simulink library "ESSLibrary"  (R2020a)
settings: Solver=VariableStepAuto  StartTime=0.0  StopTime=10.0  RelTol=1e-3
libraries: $bdroot x82, powerlib_meascontrol x10, simulink x7
(part 5 of 7)

== system ESSLibrary/Dispatch/IfActionSubsystem/Subsystem ==
  PSet : Inport
  ChargeEnableSoC : Inport  Port=2
  DischargeEnableSoC : Inport  Port=3
  AND1 : Logic  IconShape=distinctive  AllPortsSameDT=off  OutDataTypeStr=boolean
  AND2 : Logic  IconShape=distinctive  AllPortsSameDT=off  OutDataTypeStr=boolean
  Constant1 : Constant  Value=0  OutDataTypeStr=double
  IsPositive : simulink/Logic and Bit Operations/Compare To Zero  relop=>=  OutDataTypeStr=boolean
  IsPositive1 : simulink/Logic and Bit Operations/Compare To Zero  relop=<=  OutDataTypeStr=boolean
  Switch1 : Switch  Criteria=u2 ~= 0
  Switch2 : Switch  Criteria=u2 ~= 0
  P_Set : Outport
  wires:
  Constant1/1 -> Switch2/3
  PSet/1 -> Switch1/1, Switch2/1, IsPositive1/1, IsPositive/1
  IsPositive/1 -> AND1/1
  DischargeEnableSoC/1 -> AND1/2
  AND1/1 -> Switch1/2
  ChargeEnableSoC/1 -> AND2/2
  IsPositive1/1 -> AND2/1
  AND2/1 -> Switch2/2
  Switch2/1 -> Switch1/3
  Switch1/1 -> P_Set/1

== system ESSLibrary/Divider/IfActionSubsystem/Subsystem ==
  Denominator : Inport  OutDataTypeStr=double
  Compare To Zero : simulink/Logic and Bit Operations/Compare To Zero  relop===  OutDataTypeStr=boolean
  Constant : Constant  Value=0  SampleTime=-1
  Constant3 : Constant  Value=0  SampleTime=-1
  Constant4 : Constant  Value=1000  SampleTime=-1
  Sum : Sum  Inputs=|++
  Switch2 : Switch  Criteria=u2 > Threshold  Threshold=-0.00001
  Switch3 : Switch  Criteria=u2 > Threshold  Threshold=0.00001
  Switch4 : Switch  Criteria=u2 ~= 0
  Divisor : Outport  OutDataTypeStr=double
  Quality : Outport  Port=2  OutDataTypeStr=boolean
  wires:
  Constant4/1 -> Switch4/3
  Switch3/1 -> Sum/1
  Constant3/1 -> Switch2/1
  Sum/1 -> Compare To Zero/1, Switch4/2, Switch4/1
  Denominator/1 -> Switch3/2, Switch3/1, Switch2/2, Switch2/3
  Switch4/1 -> Divisor/1
  Switch2/1 -> Sum/2
  Compare To Zero/1 -> Quality/1
  Constant/1 -> Switch3/3

== system ESSLibrary/DynamicVoltWattMode/MovAvgDeltaVoltCalc/ElseMovAvgFilter ==
  Inp : Inport
  Action Port : ActionPort
  Constant : Constant  Value=0  OutDataTypeStr=int64  SampleTime=-1
  Out : Outport
  ErrorCode : Outport  Port=2
  wires:
  Constant/1 -> ErrorCode/1
  Inp/1 -> Out/1

== system ESSLibrary/DynamicVoltWattMode/MovAvgDeltaVoltCalc/IfMovAvgFilter ==
  Inp : Inport
  FilterTime : Inport  Port=2
  TimeStep : Inport  Port=3
  Action Port : ActionPort
  Constant : Constant  Value=0
  Constant1 : Constant  Value=0
  DiscreteMovingAverage : MATLAB Function  TreatAsAtomicUnit=on
  Enabled Subsystem : Subsystem  TreatAsAtomicUnit=on
  Relational Operator : RelationalOperator  Operator=>  OutDataTypeStr=boolean  ZeroCross=off  RndMeth=Simplest
  Switch : Switch  Criteria=u2 > Threshold
  Out : Outport
  ErrorCode : Outport  Port=2
  wires:
  DiscreteMovingAverage/2(ErrorCode) -> ErrorCode/1
  Constant1/1 -> Switch/3
  DiscreteMovingAverage/1(Out) -> Out/1
  TimeStep/1 -> Relational Operator/1, Enabled Subsystem/1(TimeStep)
  Relational Operator/1 -> Enabled Subsystem/Enable, Switch/2
  Enabled Subsystem/1(NoOfTimeStep) -> Switch/1
  Switch/1 -> DiscreteMovingAverage/1(NoOfTS)
  FilterTime/1 -> Enabled Subsystem/2(FilterTime)
  Constant/1 -> Relational Operator/2
  Inp/1 -> DiscreteMovingAverage/2(Inp)

== system ESSLibrary/FilterResponse/If Action Subsystem/Subsystem1 ==
  Numerator : Inport
  Denominator : Inport  Port=2
  Divide : Product  Inputs=*/
  Subsystem10 : Subsystem
  Quotient : Outport  InitialOutput=0
  Quality : Outport  Port=2  InitialOutput=0
  wires:
  Subsystem10/1(Divisor) -> Divide/2
  Divide/1 -> Quotient/1
  Denominator/1 -> Subsystem10/1(Denominator)
  Numerator/1 -> Divide/1
  Subsystem10/2(Den_Quality) -> Quality/1

== system ESSLibrary/FilterResponse/If Action Subsystem/Subsystem2 ==
  Numerator : Inport
  Denominator : Inport  Port=2
  Divide : Product  Inputs=*/
  Subsystem10 : Subsystem
  Quotient : Outport  InitialOutput=0
  Quality : Outport  Port=2  InitialOutput=0
  wires:
  Subsystem10/2(Den_Quality) -> Quality/1
  Numerator/1 -> Divide/1
  Denominator/1 -> Subsystem10/1(Denominator)
  Divide/1 -> Quotient/1
  Subsystem10/1(Divisor) -> Divide/2

== system ESSLibrary/MovAvgDeltaVoltCalc1/IfMovAvgFilter/Enabled Subsystem ==
  TimeStep : Inport
  FilterTime : Inport  Port=2
  Enable : EnablePort
  Divide : Product  Inputs=*/
  NoOfTimeStep : Outport
  wires:
  Divide/1 -> NoOfTimeStep/1
  TimeStep/1 -> Divide/2
  FilterTime/1 -> Divide/1

== system ESSLibrary/OperationModeSelector/IfAction Subsystem/Comparator ==
  note: LowerThresholdID
  note: UpperThresholdID
  note: CategoryID = 1
  Enable/Disable : Inport
  "Input " : Inport  Port=2
  UpperTrhd : Inport  Port=3
  LowerTrhd : Inport  Port=4
  HystSelection : Inport  Port=5
  AbsHyst : Inport  Port=6
  RelHyst : Inport  Port=7
  VariableIdentifier : Inport  Port=8
  Basic alarm ver2.0 : Subsystem
  CategoryID : Constant  OutDataTypeStr=int64
  Constant1 : Constant  OutDataTypeStr=int64
  Constant10 : Constant  Value=0  OutDataTypeStr=int64
  Constant11 : Constant  Value=0  OutDataTypeStr=int64
  Constant2 : Constant  Value=2  OutDataTypeStr=int64
  Gain : Gain  Gain=100
  Gain1 : Gain  Gain=10000
  Sum : Sum  Inputs=+++  OutDataTypeStr=int64
  Switch1 : Switch  Criteria=u2 ~= 0  OutDataTypeStr=int64
  Switch2 : Switch  Criteria=u2 ~= 0  OutDataTypeStr=int64
  Switch3 : Switch  Criteria=u2 ~= 0  OutDataTypeStr=int64
  Terminator1 : Terminator
  ErrorCode : Outport
  MaxLimitCrossed : Outport  Port=2
  MinLimitCrossed : Outport  Port=3
  wires:
  Basic alarm ver2.0/1(MaxLimitCrossed) -> MaxLimitCrossed/1, Switch1/2
  Constant2/1 -> Switch2/1
  CategoryID/1 -> Gain/1
  Switch1/1 -> Switch3/2, Sum/1
  Constant1/1 -> Switch1/1
  Constant11/1 -> Switch2/3
  HystSelection/1 -> Basic alarm ver2.0/5(HystSelection)
  Basic alarm ver2.0/2(MinLimitCrossed) -> MinLimitCrossed/1, Switch2/2
  Constant10/1 -> Switch3/3
  Basic alarm ver2.0/3(ErrorCode) -> Terminator1/1
  Sum/1 -> Switch3/1
  "Input "/1 -> Basic alarm ver2.0/2("Input ")
  Switch2/1 -> Switch1/3
  VariableIdentifier/1 -> Gain1/1
  AbsHyst/1 -> Basic alarm ver2.0/6(AbsHyst)
  RelHyst/1 -> Basic alarm ver2.0/7(RelHyst)
  Enable/Disable/1 -> Basic alarm ver2.0/1(Enable/disable)
  Switch3/1 -> ErrorCode/1
  UpperTrhd/1 -> Basic alarm ver2.0/3(UpperTrhd)
  LowerTrhd/1 -> Basic alarm ver2.0/4(LowerTrhd)
  Gain/1 -> Sum/2
  Gain1/1 -> Sum/3

== system ESSLibrary/PFReference_P/If Action Subsystem/Basic alarm ver1.0 ==
  Enable/disable : Inport  OutDataTypeStr=boolean
  "Input " : Inport  Port=2
  UpperTrhd : Inport  Port=3
  LowerTrhd : Inport  Port=4
  HystSelection : Inport  Port=5  OutDataTypeStr=int32
  AbsHyst : Inport  Port=6
  RelHyst : Inport  Port=7
  Enable/disable1 : InportShadow  OutDataTypeStr=boolean
  Enabled Subsystem : Subsystem  TreatAsAtomicUnit=on
  Enabled Subsystem1 : Subsystem  TreatAsAtomicUnit=on
  If : If  IfExpression=u1 ~=0
  Switch : Switch  Criteria=u2 > Threshold
  Switch3 : Switch  Criteria=u2 > Threshold
  "Output " : Outport
  ErrorCode : Outport  Port=2
  wires:
  HystSelection/1 -> Enabled Subsystem1/4(HystSelection)
  RelHyst/1 -> Enabled Subsystem1/6(RelHyst)
  AbsHyst/1 -> Enabled Subsystem1/5(AbsHyst)
  LowerTrhd/1 -> Enabled Subsystem1/3(LowerTrhd)
  UpperTrhd/1 -> Enabled Subsystem1/2(UpperTrhd)
  "Input "/1 -> Enabled Subsystem1/1("Input ")
  Enable/disable1/1 -> Switch3/2, Switch/2
  [Else_Logx_value] -> Switch/3
  Switch/1 -> "Output "/1
  Enabled Subsystem1/1("Output ") -> [If_Logx_value]
  [Elase_Errorcode] -> Switch3/3
  [If_Errorcode] -> Switch3/1
  [If_Logx_value] -> Switch/1
  Enabled Subsystem/1("Output ") -> [Else_Logx_value]
  Enabled Subsystem/2(ErrorCode) -> [Elase_Errorcode]
  Switch3/1 -> ErrorCode/1
  Enabled Subsystem1/2(ErrorCode) -> [If_Errorcode]
  If/1 -> Enabled Subsystem1/Action
  If/2 -> Enabled Subsystem/Action
  Enable/disable/1 -> If/1

== system ESSLibrary/PFReference_P/If Action Subsystem/Safe Divider ==
  Enable : Inport  OutDataTypeStr=boolean
  Numerator : Inport  Port=2  OutDataTypeStr=double
  Denominator : Inport  Port=3  OutDataTypeStr=double
  Abs : Abs
  If : If  IfExpression=u1 ~= 0
  Subsystem : Subsystem
  Subsystem1 : Subsystem
  Switch1 : Switch  Criteria=u2 ~= 0
  Switch6 : Switch  Criteria=u2 > Threshold
  Switch7 : Switch  Criteria=u2 > Threshold
  Switch8 : Switch  Criteria=u2 > Threshold
  Quotient : Outport  OutDataTypeStr=double
  Quality : Outport  Port=2  OutDataTypeStr=boolean
  ErrorCode : Outport  Port=3  OutDataTypeStr=int64
  wires:
  If/2 -> Subsystem1/Action
  [Quotient] -> Switch1/2, Switch1/1
  Switch6/1 -> Quality/1
  [DivErrorCode] -> Switch8/1
  Subsystem1/3(Out5) -> [DivErrorCodeD]
  Switch8/1 -> ErrorCode/1
  Subsystem/2(Out) -> [Quotient]
  [QuotientD] -> Switch7/3
  Denominator/1 -> [Denom]
  Switch7/1 -> Quotient/1
  [DivErrorCodeD] -> Switch8/3
  Subsystem1/1(Out3) -> [QualityD]
  Switch1/1 -> Switch7/1
  Subsystem/1(Quality) -> [Quality]
  If/1 -> Subsystem/Action
  Subsystem1/2(Out4) -> [QuotientD]
  [Denom] -> Subsystem/2(Denominator)
  Numerator/1 -> [Num]
  Subsystem/3(ErrorCode) -> [DivErrorCode]
  [Quotient] -> Abs/1
  [Num] -> Subsystem1/1(In1)
  [QualityD] -> Switch6/3
  Enable/1 -> If/1, Switch6/2, Switch7/2, Switch8/2
  Abs/1 -> Switch1/3
  [Num] -> Subsystem/1(Numerator)
  [Quality] -> Switch6/1

== system ESSLibrary/QReference_PF/If Action Subsystem/Subsystem1 ==
  PF : Inport
  PFSign : Inport  Port=2
  PMeas : Inport  Port=3
  Constant : Constant  OutDataTypeStr=boolean
  Constant1 : Constant
  Constant9 : Constant  Value=-1  OutDataTypeStr=double  SampleTime=-1
  Divide : Product  Inputs=**
  Divide3 : Product  Inputs=**
  Safe Divider : Subsystem  Description=|
      | This function divides input values accounting for a predefined dead band for denominator to avoid occurrence of divide by zero condition. 
      | If the input for denominator is inside the dead band then the function returns predefined output with quality bit as one. 
      | If input value for denominator is in the normal range, the function returns the calculated quotient with quality bit as zero.
  Square : Math  Operator=square  SaturateOnIntegerOverflow=on
  Square Root : Sqrt  SaturateOnIntegerOverflow=on
  Sum : Sum  Inputs=+-
  Switch2 : Switch  Criteria=u2 > Threshold
  Terminator2 : Terminator
  QOut : Outport
  ErrorCode : Outport  Port=2
  wires:
  Switch2/1 -> QOut/1
  PMeas/1 -> Divide/1
  Constant9/1 -> Divide3/2
  Safe Divider/1(Quotient) -> Divide/2
  PFSign/1 -> Switch2/2
  Divide/1 -> Divide3/1, Switch2/1
  Square Root/1 -> Safe Divider/2(Numerator)
  Square/1 -> Sum/2
  PF/1 -> Safe Divider/3(Denominator), Square/1
  Sum/1 -> Square Root/1
  Constant1/1 -> Sum/1
  Safe Divider/2(Quality) -> Terminator2/1
  Constant/1 -> Safe Divider/1(Enable)
  Divide3/1 -> Switch2/3
  Safe Divider/3(ErrorCode) -> ErrorCode/1

== system ESSLibrary/SoCManagement/IfActionSubsystem/Comparator ==
  note: CategoryID = 1
  note: UpperThresholdID
  note: LowerThresholdID
  Enable/Disable : Inport
  "Input " : Inport  Port=2
  UpperTrhd : Inport  Port=3
  LowerTrhd : Inport  Port=4
  HystSelection : Inport  Port=5
  AbsHyst : Inport  Port=6
  RelHyst : Inport  Port=7
  VariableIdentifier : Inport  Port=8
  Basic alarm ver2.0 : Subsystem
  CategoryID : Constant  OutDataTypeStr=int64
  Constant1 : Constant  OutDataTypeStr=int64
  Constant10 : Constant  Value=0  OutDataTypeStr=int64
  Constant11 : Constant  Value=0  OutDataTypeStr=int64
  Constant2 : Constant  Value=2  OutDataTypeStr=int64
  Gain : Gain  Gain=100
  Gain1 : Gain  Gain=10000
  Sum : Sum  Inputs=+++  OutDataTypeStr=int64
  Switch1 : Switch  Criteria=u2 ~= 0  OutDataTypeStr=int64
  Switch2 : Switch  Criteria=u2 ~= 0  OutDataTypeStr=int64
  Switch3 : Switch  Criteria=u2 ~= 0  OutDataTypeStr=int64
  Terminator1 : Terminator
  ErrorCode : Outport
  MaxLimitCrossed : Outport  Port=2
  MinLimitCrossed : Outport  Port=3
  wires:
  Gain1/1 -> Sum/3
  Gain/1 -> Sum/2
  LowerTrhd/1 -> Basic alarm ver2.0/4(LowerTrhd)
  UpperTrhd/1 -> Basic alarm ver2.0/3(UpperTrhd)
  Switch3/1 -> ErrorCode/1
  Enable/Disable/1 -> Basic alarm ver2.0/1(Enable/disable)
  RelHyst/1 -> Basic alarm ver2.0/7(RelHyst)
  AbsHyst/1 -> Basic alarm ver2.0/6(AbsHyst)
  VariableIdentifier/1 -> Gain1/1
  Switch2/1 -> Switch1/3
  "Input "/1 -> Basic alarm ver2.0/2("Input ")
  Sum/1 -> Switch3/1
  Basic alarm ver2.0/3(ErrorCode) -> Terminator1/1
  Constant10/1 -> Switch3/3
  Basic alarm ver2.0/2(MinLimitCrossed) -> Switch2/2, MinLimitCrossed/1
  HystSelection/1 -> Basic alarm ver2.0/5(HystSelection)
  Constant11/1 -> Switch2/3
  Constant1/1 -> Switch1/1
  Switch1/1 -> Sum/1, Switch3/2
  CategoryID/1 -> Gain/1
  Constant2/1 -> Switch2/1
  Basic alarm ver2.0/1(MaxLimitCrossed) -> Switch1/2, MaxLimitCrossed/1

== system ESSLibrary/ActivePowerSmoothing/MovAvgDeltaVoltCalc/IfMovAvgFilter/Enabled Subsystem ==
  TimeStep : Inport
  FilterTime : Inport  Port=2
  Enable : EnablePort
  Divide : Product  Inputs=*/
  NoOfTimeStep : Outport
  wires:
  Divide/1 -> NoOfTimeStep/1
  TimeStep/1 -> Divide/2
  FilterTime/1 -> Divide/1

== system ESSLibrary/ChargeDischargeStorageMode/Comparator/Basic alarm ver2.0/Enabled Subsystem ==
  Action Port : ActionPort
  Constant3 : Constant  Value=0  OutDataTypeStr=boolean  SampleTime=-1
  "MaxLimitCrossed " : Outport
  ErrorCode : Outport  Port=2
  MinLimitCrossed : Outport  Port=3
  wires:
  Constant3/1 -> ErrorCode/1, MinLimitCrossed/1, "MaxLimitCrossed "/1

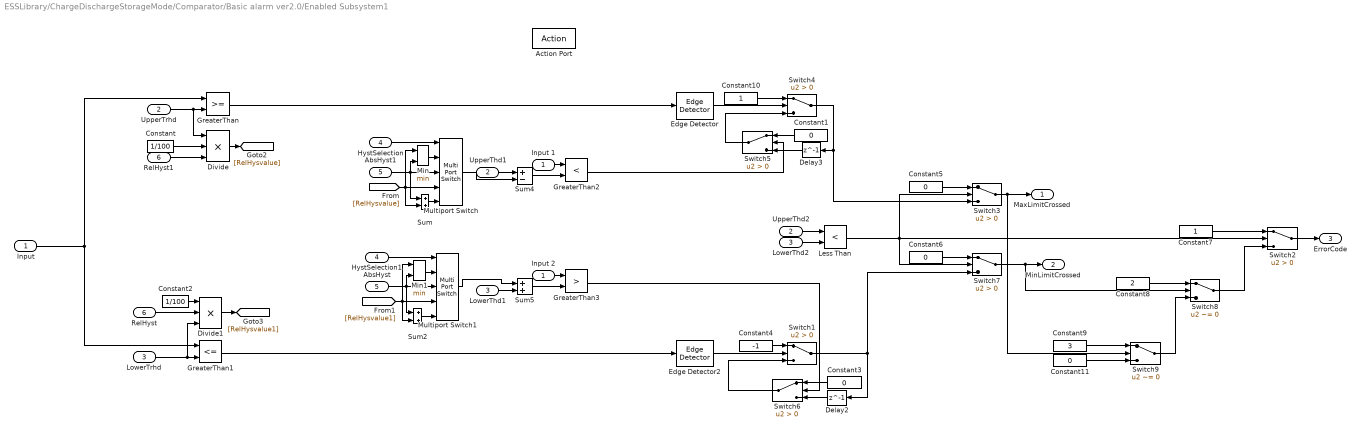
== system ESSLibrary/ChargeDischargeStorageMode/Comparator/Basic alarm ver2.0/Enabled Subsystem1 ==
  "Input " : Inport
  UpperTrhd : Inport  Port=2
  LowerTrhd : Inport  Port=3
  HystSelection : Inport  Port=4
  AbsHyst : Inport  Port=5
  RelHyst : Inport  Port=6
  Action Port : ActionPort
  AbsHyst1 : InportShadow  Port=5
  Constant : Constant  Value=1/100  SampleTime=-1
  Constant1 : Constant  Value=0  OutDataTypeStr=int8  SampleTime=-1
  Constant10 : Constant  OutDataTypeStr=int8  SampleTime=-1
  Constant11 : Constant  Value=0  OutDataTypeStr=int64  SampleTime=-1
  Constant2 : Constant  Value=1/100  SampleTime=-1
  Constant3 : Constant  Value=0  OutDataTypeStr=int8  SampleTime=-1
  Constant4 : Constant  Value=-1  OutDataTypeStr=int8  SampleTime=-1
  Constant5 : Constant  Value=0  OutDataTypeStr=boolean  SampleTime=-1
  Constant6 : Constant  Value=0  OutDataTypeStr=boolean  SampleTime=-1
  Constant7 : Constant  OutDataTypeStr=int64  SampleTime=-1
  Constant8 : Constant  Value=2  OutDataTypeStr=int64  SampleTime=-1
  Constant9 : Constant  Value=3  OutDataTypeStr=int64  SampleTime=-1
  Delay2 : Delay  DelayLength=1  InitialCondition=0
  Delay3 : Delay  DelayLength=1  InitialCondition=0
  Divide : Product  Inputs=***
  Divide1 : Product  Inputs=***
  Edge Detector : powerlib_meascontrol/Logic/Edge Detector  model=Rising  ic=0  Ts=-1
      settings: SourceProductBaseCode=PS
  Edge Detector2 : powerlib_meascontrol/Logic/Edge Detector  model=Rising  ic=0  Ts=-1
      settings: SourceProductBaseCode=PS
  GreaterThan : RelationalOperator  OutDataTypeStr=boolean  RndMeth=Simplest
  GreaterThan1 : RelationalOperator  Operator=<=  OutDataTypeStr=boolean  RndMeth=Simplest
  GreaterThan2 : RelationalOperator  Operator=<  OutDataTypeStr=boolean  RndMeth=Simplest
  GreaterThan3 : RelationalOperator  Operator=>  OutDataTypeStr=boolean  RndMeth=Simplest
  HystSelection1 : InportShadow  Port=4
  Input 1 : InportShadow
  Input 2 : InportShadow
  Less Than : RelationalOperator  Operator=<  OutDataTypeStr=boolean  RndMeth=Simplest
  LowerThd1 : InportShadow  Port=3
  LowerThd2 : InportShadow  Port=3
  Min : MinMax  Inputs=2
  Min1 : MinMax  Inputs=2
  Multiport Switch : MultiPortSwitch  Inputs=4
  Multiport Switch1 : MultiPortSwitch  Inputs=4
  RelHyst1 : InportShadow  Port=6
  Sum : Sum
  Sum2 : Sum
  Sum4 : Sum  Inputs=+-
  Sum5 : Sum
  Switch{1..7} (7 alike) : Switch  Criteria=u2 > Threshold
  Switch8 : Switch  Criteria=u2 ~= 0
  Switch9 : Switch  Criteria=u2 ~= 0
  UpperThd1 : InportShadow  Port=2
  UpperThd2 : InportShadow  Port=2
  MaxLimitCrossed : Outport
  MinLimitCrossed : Outport  Port=2
  ErrorCode : Outport  Port=3  OutDataTypeStr=int64
  wires:
  Constant4/1 -> Switch1/1
  GreaterThan/1 -> Edge Detector/1
  "Input "/1 -> GreaterThan/1, GreaterThan1/1
  UpperTrhd/1 -> Divide/1, GreaterThan/2
  LowerTrhd/1 -> Divide1/3, GreaterThan1/2
  HystSelection/1 -> Multiport Switch/1
  AbsHyst1/1 -> Min/2, Sum/1, Multiport Switch/3
  [RelHysvalue] -> Min/1, Sum/2, Multiport Switch/4
  Sum/1 -> Multiport Switch/5
  Divide/1 -> [RelHysvalue]
  Min/1 -> Multiport Switch/2
  Input 1/1 -> GreaterThan2/1
  Constant10/1 -> Switch4/1
  Edge Detector/1 -> Switch4/2
  Switch5/1 -> Switch4/3
  Switch4/1 -> Switch3/3, Delay3/1
  Constant/1 -> Divide/2
  RelHyst1/1 -> Divide/3
  RelHyst/1 -> Divide1/2
  Constant2/1 -> Divide1/1
  Divide1/1 -> [RelHysvalue1]
  HystSelection1/1 -> Multiport Switch1/1
  Min1/1 -> Multiport Switch1/2
  AbsHyst/1 -> Sum2/1, Min1/2, Multiport Switch1/3
  [RelHysvalue1] -> Sum2/2, Multiport Switch1/4, Min1/1
  Sum2/1 -> Multiport Switch1/5
  Input 2/1 -> GreaterThan3/1
  GreaterThan1/1 -> Edge Detector2/1
  Edge Detector2/1 -> Switch1/2
  Switch6/1 -> Switch1/3
  GreaterThan3/1 -> Switch6/2
  Sum4/1 -> GreaterThan2/2
  Multiport Switch/1 -> Sum4/2
  UpperThd1/1 -> Sum4/1
  Sum5/1 -> GreaterThan3/2
  Multiport Switch1/1 -> Sum5/1
  LowerThd1/1 -> Sum5/2
  GreaterThan2/1 -> Switch5/2
  Constant1/1 -> Switch5/1
  Constant3/1 -> Switch6/1
  Delay3/1 -> Switch5/3
  Delay2/1 -> Switch6/3
  Switch3/1 -> Switch9/2, MaxLimitCrossed/1
  Less Than/1 -> Switch2/2, Switch3/2, Switch7/2
  Constant5/1 -> Switch3/1
  Switch1/1 -> Switch7/3, Delay2/1
  Constant6/1 -> Switch7/1
  Switch7/1 -> Switch8/2, MinLimitCrossed/1
  Switch8/1 -> Switch2/3
  Constant7/1 -> Switch2/1
  Switch2/1 -> ErrorCode/1
  LowerThd2/1 -> Less Than/2
  UpperThd2/1 -> Less Than/1
  Constant8/1 -> Switch8/1
  Constant9/1 -> Switch9/1
  Constant11/1 -> Switch9/3
  Switch9/1 -> Switch8/3

== system ESSLibrary/Dispatch/IfActionSubsystem/PrioritySelector/ActivePowerPriority ==
  "EnablePQCapabilityCurve " : Inport
  Pcapability1 : Inport  Port=2
  Pcapability2 : Inport  Port=3
  Pcapability3 : Inport  Port=4
  Pcapability4 : Inport  Port=5
  Pcapability5 : Inport  Port=6
  Pcapability6 : Inport  Port=7
  Pcapability7 : Inport  Port=8
  Pcapability8 : Inport  Port=9
  Qcapability1 : Inport  Port=10
  Qcapability2 : Inport  Port=11
  Qcapability3 : Inport  Port=12
  Qcapability4 : Inport  Port=13
  Qcapability5 : Inport  Port=14
  Qcapability6 : Inport  Port=15
  Qcapability7 : Inport  Port=16
  Qcapability8 : Inport  Port=17
  ECPAppPow : Inport  Port=18
  EnablePFLimit : Inport  Port=19
  PFOperMax : Inport  Port=20
  PFOperMin : Inport  Port=21
  ActivePowerCalc : Inport  Port=22
  ReactivePowerCalc : Inport  Port=23
  Action Port : ActionPort  ActionPortLabel=else
  ActivePowerCalc1 : InportShadow  Port=22
  ActivePowerPriority_NoPQCurve : Subsystem  TreatAsAtomicUnit=on
  ActivePowerPriority_PQCurve : Subsystem  TreatAsAtomicUnit=on
  ECPAppPow1 : InportShadow  Port=18
  EnablePFLimit1 : InportShadow  Port=19
  If : If  IfExpression=u1 == 1
  Merge : Merge
  Merge1 : Merge
  PFOperMax1 : InportShadow  Port=20
  PFOperMin1 : InportShadow  Port=21
  ReactivePowerCalc1 : InportShadow  Port=23
  ActivePowerOut : Outport
  ReactivePowerOut : Outport  Port=2
  wires:
  "EnablePQCapabilityCurve "/1 -> If/1
  If/1 -> ActivePowerPriority_PQCurve/Action
  If/2 -> ActivePowerPriority_NoPQCurve/Action
  Pcapability1/1 -> ActivePowerPriority_PQCurve/1(Pcapability1)
  Pcapability2/1 -> ActivePowerPriority_PQCurve/2(Pcapability2)
  Pcapability3/1 -> ActivePowerPriority_PQCurve/3(Pcapability3)
  Pcapability4/1 -> ActivePowerPriority_PQCurve/4(Pcapability4)
  Pcapability5/1 -> ActivePowerPriority_PQCurve/5(Pcapability5)
  Pcapability6/1 -> ActivePowerPriority_PQCurve/6(Pcapability6)
  Pcapability7/1 -> ActivePowerPriority_PQCurve/7(Pcapability7)
  Pcapability8/1 -> ActivePowerPriority_PQCurve/8(Pcapability8)
  Qcapability1/1 -> ActivePowerPriority_PQCurve/9(Qcapability1)
  Qcapability2/1 -> ActivePowerPriority_PQCurve/10(Qcapability2)
  Qcapability3/1 -> ActivePowerPriority_PQCurve/11(Qcapability3)
  Qcapability4/1 -> ActivePowerPriority_PQCurve/12(Qcapability4)
  Qcapability5/1 -> ActivePowerPriority_PQCurve/13(Qcapability5)
  Qcapability6/1 -> ActivePowerPriority_PQCurve/14(Qcapability6)
  Qcapability7/1 -> ActivePowerPriority_PQCurve/15(Qcapability7)
  Qcapability8/1 -> ActivePowerPriority_PQCurve/16(Qcapability8)
  ECPAppPow/1 -> ActivePowerPriority_PQCurve/17(ECPAppPow)
  EnablePFLimit/1 -> ActivePowerPriority_PQCurve/18(EnablePFLimit)
  PFOperMax/1 -> ActivePowerPriority_PQCurve/19(PFOperMax)
  PFOperMin/1 -> ActivePowerPriority_PQCurve/20(PFOperMin)
  ActivePowerCalc/1 -> ActivePowerPriority_PQCurve/21(ActivePowerCalc)
  ReactivePowerCalc/1 -> ActivePowerPriority_PQCurve/22(ReactivePowerCalc)
  ActivePowerPriority_NoPQCurve/1(ActivePowerOut) -> [ActivePowerPriority_NoPQCurveActivePowerOut]
  ActivePowerPriority_NoPQCurve/2(ReactivePowerOut) -> [ActivePowerPriority_NoPQCurveReactivePowerOut]
  ActivePowerPriority_PQCurve/1(ActivePowerOut) -> [ActivePowerPriority_PQCurveActivePowerOut]
  ActivePowerPriority_PQCurve/2(ReactivePowerOut) -> [ActivePowerPriority_PQCurveReactivePowerOut]
  [ActivePowerPriority_NoPQCurveActivePowerOut] -> Merge/1
  [ActivePowerPriority_PQCurveActivePowerOut] -> Merge/2
  [ActivePowerPriority_NoPQCurveReactivePowerOut] -> Merge1/1
  [ActivePowerPriority_PQCurveReactivePowerOut] -> Merge1/2
  Merge/1 -> ActivePowerOut/1
  Merge1/1 -> ReactivePowerOut/1
  ActivePowerCalc1/1 -> ActivePowerPriority_NoPQCurve/1(ActivePowerCalc)
  ECPAppPow1/1 -> ActivePowerPriority_NoPQCurve/3(ECPAppPow)
  ReactivePowerCalc1/1 -> ActivePowerPriority_NoPQCurve/2(ReactivePowerCalc)
  EnablePFLimit1/1 -> ActivePowerPriority_NoPQCurve/4(EnablePFLimit)
  PFOperMax1/1 -> ActivePowerPriority_NoPQCurve/5(PFOperMax)
  PFOperMin1/1 -> ActivePowerPriority_NoPQCurve/6(PFOperMin)

== system ESSLibrary/Dispatch/IfActionSubsystem/PrioritySelector/ReactivePowerPriority ==
  "EnablePQCapabilityCurve " : Inport
  Pcapability1 : Inport  Port=2
  Pcapability2 : Inport  Port=3
  Pcapability3 : Inport  Port=4
  Pcapability4 : Inport  Port=5
  Pcapability5 : Inport  Port=6
  Pcapability6 : Inport  Port=7
  Pcapability7 : Inport  Port=8
  Pcapability8 : Inport  Port=9
  Qcapability1 : Inport  Port=10
  Qcapability2 : Inport  Port=11
  Qcapability3 : Inport  Port=12
  Qcapability4 : Inport  Port=13
  Qcapability5 : Inport  Port=14
  Qcapability6 : Inport  Port=15
  Qcapability7 : Inport  Port=16
  Qcapability8 : Inport  Port=17
  ECPAppPow : Inport  Port=18
  EnablePFLimit : Inport  Port=19
  PFOperMax : Inport  Port=20
  PFOperMin : Inport  Port=21
  ActivePowerCalc : Inport  Port=22
  ReactivePowerCalc : Inport  Port=23
  Action Port : ActionPort  ActionPortLabel=if(u1 == 2)
  ActivePowerCalc1 : InportShadow  Port=22
  ECPAppPow1 : InportShadow  Port=18
  EnablePFLimit1 : InportShadow  Port=19
  If : If  IfExpression=u1 == 1
  Merge : Merge
  Merge1 : Merge
  PFOperMax1 : InportShadow  Port=20
  PFOperMin1 : InportShadow  Port=21
  ReactivePowerCalc1 : InportShadow  Port=23
  ReactivePowerPriority_NoPQCurve : Subsystem  TreatAsAtomicUnit=on
  ReactivePowerPriority_PQCurve : Subsystem  TreatAsAtomicUnit=on
  ActivePowerOut : Outport
  ReactivePowerOut : Outport  Port=2
  wires:
  "EnablePQCapabilityCurve "/1 -> If/1
  If/1 -> ReactivePowerPriority_PQCurve/Action
  If/2 -> ReactivePowerPriority_NoPQCurve/Action
  Pcapability1/1 -> ReactivePowerPriority_PQCurve/1(Pcapability1)
  Pcapability2/1 -> ReactivePowerPriority_PQCurve/2(Pcapability2)
  Pcapability3/1 -> ReactivePowerPriority_PQCurve/3(Pcapability3)
  Pcapability4/1 -> ReactivePowerPriority_PQCurve/4(Pcapability4)
  Pcapability5/1 -> ReactivePowerPriority_PQCurve/5(Pcapability5)
  Pcapability6/1 -> ReactivePowerPriority_PQCurve/6(Pcapability6)
  Pcapability7/1 -> ReactivePowerPriority_PQCurve/7(Pcapability7)
  Pcapability8/1 -> ReactivePowerPriority_PQCurve/8(Pcapability8)
  Qcapability1/1 -> ReactivePowerPriority_PQCurve/9(Qcapability1)
  Qcapability2/1 -> ReactivePowerPriority_PQCurve/10(Qcapability2)
  Qcapability3/1 -> ReactivePowerPriority_PQCurve/11(Qcapability3)
  Qcapability4/1 -> ReactivePowerPriority_PQCurve/12(Qcapability4)
  Qcapability5/1 -> ReactivePowerPriority_PQCurve/13(Qcapability5)
  Qcapability6/1 -> ReactivePowerPriority_PQCurve/14(Qcapability6)
  Qcapability7/1 -> ReactivePowerPriority_PQCurve/15(Qcapability7)
  Qcapability8/1 -> ReactivePowerPriority_PQCurve/16(Qcapability8)
  ECPAppPow/1 -> ReactivePowerPriority_PQCurve/17(ECPAppPow)
  EnablePFLimit/1 -> ReactivePowerPriority_PQCurve/18(EnablePFLimit)
  PFOperMax/1 -> ReactivePowerPriority_PQCurve/19(PFOperMax)
  PFOperMin/1 -> ReactivePowerPriority_PQCurve/20(PFOperMin)
  ActivePowerCalc/1 -> ReactivePowerPriority_PQCurve/21(ActivePowerCalc)
  ReactivePowerCalc/1 -> ReactivePowerPriority_PQCurve/22(ReactivePowerCalc)
  ReactivePowerPriority_NoPQCurve/1(ActivePowerOut) -> [ActivePowerPriority_NoPQCurveActivePowerOut]
  ReactivePowerPriority_NoPQCurve/2(ReactivePowerOut) -> [ActivePowerPriority_NoPQCurveReactivePowerOut]
  ReactivePowerPriority_PQCurve/1(ActivePowerOut) -> [ActivePowerPriority_PQCurveActivePowerOut]
  ReactivePowerPriority_PQCurve/2(ReactivePowerOut) -> [ActivePowerPriority_PQCurveReactivePowerOut]
  [ActivePowerPriority_NoPQCurveActivePowerOut] -> Merge/1
  [ActivePowerPriority_PQCurveActivePowerOut] -> Merge/2
  [ActivePowerPriority_NoPQCurveReactivePowerOut] -> Merge1/1
  [ActivePowerPriority_PQCurveReactivePowerOut] -> Merge1/2
  Merge/1 -> ActivePowerOut/1
  Merge1/1 -> ReactivePowerOut/1
  ActivePowerCalc1/1 -> ReactivePowerPriority_NoPQCurve/1(ActivePowerCalc)
  ECPAppPow1/1 -> ReactivePowerPriority_NoPQCurve/3(ECPAppPow)
  ReactivePowerCalc1/1 -> ReactivePowerPriority_NoPQCurve/2(ReactivePowerCalc)
  EnablePFLimit1/1 -> ReactivePowerPriority_NoPQCurve/4(EnablePFLimit)
  PFOperMax1/1 -> ReactivePowerPriority_NoPQCurve/5(PFOperMax)
  PFOperMin1/1 -> ReactivePowerPriority_NoPQCurve/6(PFOperMin)

== system ESSLibrary/DynamicVoltWattMode/MovAvgDeltaVoltCalc/IfMovAvgFilter/Enabled Subsystem ==
  TimeStep : Inport
  FilterTime : Inport  Port=2
  Enable : EnablePort
  Divide : Product  Inputs=*/
  NoOfTimeStep : Outport
  wires:
  FilterTime/1 -> Divide/1
  TimeStep/1 -> Divide/2
  Divide/1 -> NoOfTimeStep/1

== system ESSLibrary/FilterResponse/If Action Subsystem/Subsystem1/Subsystem10 ==
  Denominator : Inport
  Compare To Zero : simulink/Logic and Bit Operations/Compare To Zero  relop===  OutDataTypeStr=boolean
  Constant4 : Constant  SampleTime=-1
  Switch3 : Switch  Criteria=u2 ~= 0
  Divisor : Outport
  Den_Quality : Outport  Port=2
  wires:
  Denominator/1 -> Switch3/1, Switch3/2, Compare To Zero/1
  Switch3/1 -> Divisor/1
  Compare To Zero/1 -> Den_Quality/1
  Constant4/1 -> Switch3/3

== system ESSLibrary/FilterResponse/If Action Subsystem/Subsystem2/Subsystem10 ==
  Denominator : Inport
  Compare To Zero : simulink/Logic and Bit Operations/Compare To Zero  relop===  OutDataTypeStr=boolean
  Constant4 : Constant  SampleTime=-1
  Switch3 : Switch  Criteria=u2 ~= 0
  Divisor : Outport
  Den_Quality : Outport  Port=2
  wires:
  Constant4/1 -> Switch3/3
  Compare To Zero/1 -> Den_Quality/1
  Switch3/1 -> Divisor/1
  Denominator/1 -> Compare To Zero/1, Switch3/2, Switch3/1

== system ESSLibrary/OperationModeSelector/IfAction Subsystem/Comparator/Basic alarm ver2.0 ==
  Enable/disable : Inport  OutDataTypeStr=boolean
  "Input " : Inport  Port=2
  UpperTrhd : Inport  Port=3
  LowerTrhd : Inport  Port=4
  HystSelection : Inport  Port=5  OutDataTypeStr=int32
  AbsHyst : Inport  Port=6
  RelHyst : Inport  Port=7
  Enable/disable1 : InportShadow  OutDataTypeStr=boolean
  Enabled Subsystem : Subsystem  TreatAsAtomicUnit=on
  Enabled Subsystem1 : Subsystem  TreatAsAtomicUnit=on
  If : If  IfExpression=u1 ~=0
  Switch : Switch  Criteria=u2 > Threshold
  Switch1 : Switch  Criteria=u2 > Threshold
  Switch3 : Switch  Criteria=u2 > Threshold
  MaxLimitCrossed : Outport  OutDataTypeStr=boolean
  MinLimitCrossed : Outport  Port=2  OutDataTypeStr=boolean
  ErrorCode : Outport  Port=3  OutDataTypeStr=int64
  wires:
  Enable/disable/1 -> If/1
  If/2 -> Enabled Subsystem/Action
  If/1 -> Enabled Subsystem1/Action
  Enabled Subsystem1/3(ErrorCode) -> [If_Errorcode]
  Enabled Subsystem/2(ErrorCode) -> [Else_Errorcode]
  Enabled Subsystem/1("MaxLimitCrossed ") -> [Else_MaxLimitCrossed]
  [If_MaxLimitCrossed] -> Switch/1
  [If_Errorcode] -> Switch3/1
  [Else_Errorcode] -> Switch3/3
  Enabled Subsystem1/1(MaxLimitCrossed) -> [If_MaxLimitCrossed]
  Switch/1 -> MaxLimitCrossed/1
  [Else_MaxLimitCrossed] -> Switch/3
  Enable/disable1/1 -> Switch3/2, Switch1/2, Switch/2
  "Input "/1 -> Enabled Subsystem1/1("Input ")
  UpperTrhd/1 -> Enabled Subsystem1/2(UpperTrhd)
  LowerTrhd/1 -> Enabled Subsystem1/3(LowerTrhd)
  AbsHyst/1 -> Enabled Subsystem1/5(AbsHyst)
  RelHyst/1 -> Enabled Subsystem1/6(RelHyst)
  HystSelection/1 -> Enabled Subsystem1/4(HystSelection)
  Enabled Subsystem1/2(MinLimitCrossed) -> [If_MinLimitCrossed]
  Enabled Subsystem/3(MinLimitCrossed) -> [Else_MinLimitCrossed]
  [If_MinLimitCrossed] -> Switch1/1
  [Else_MinLimitCrossed] -> Switch1/3
  Switch1/1 -> MinLimitCrossed/1
  Switch3/1 -> ErrorCode/1

== system ESSLibrary/PFReference_P/If Action Subsystem/Basic alarm ver1.0/Enabled Subsystem ==
  Action Port : ActionPort
  Constant2 : Constant  Value=00000000000009  OutDataTypeStr=int32
  Constant3 : Constant  Value=0  OutDataTypeStr=double
  "Output " : Outport
  ErrorCode : Outport  Port=2
  wires:
  Constant3/1 -> "Output "/1
  Constant2/1 -> ErrorCode/1

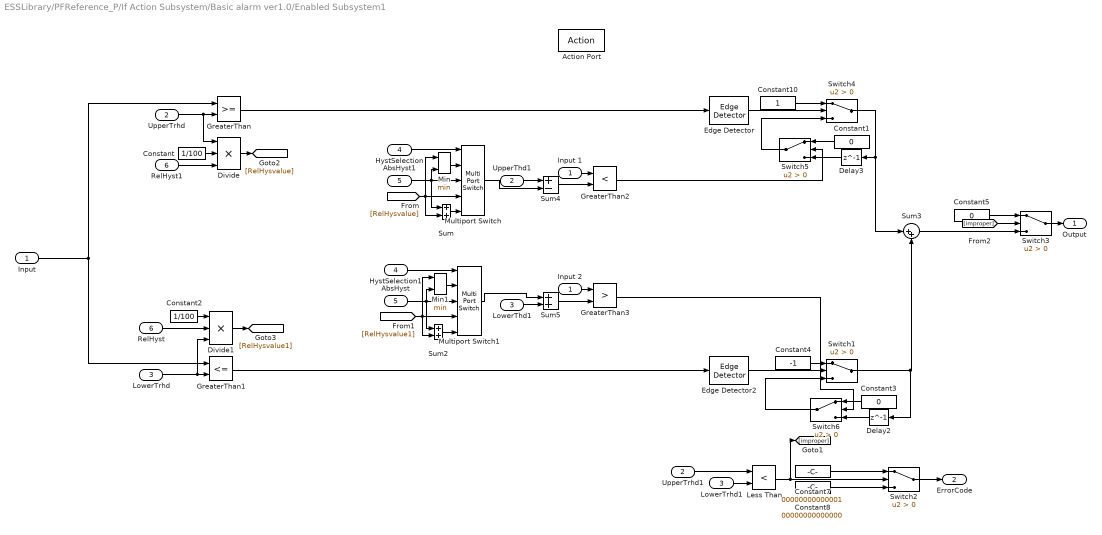
== system ESSLibrary/PFReference_P/If Action Subsystem/Basic alarm ver1.0/Enabled Subsystem1 ==
  "Input " : Inport
  UpperTrhd : Inport  Port=2
  LowerTrhd : Inport  Port=3
  HystSelection : Inport  Port=4
  AbsHyst : Inport  Port=5
  RelHyst : Inport  Port=6
  Action Port : ActionPort
  AbsHyst1 : InportShadow  Port=5
  Constant : Constant  Value=1/100  SampleTime=-1
  Constant1 : Constant  Value=0  OutDataTypeStr=int32  SampleTime=-1
  Constant10 : Constant  OutDataTypeStr=int32  SampleTime=-1
  Constant2 : Constant  Value=1/100  SampleTime=-1
  Constant3 : Constant  Value=0  OutDataTypeStr=int32  SampleTime=-1
  Constant4 : Constant  Value=-1  OutDataTypeStr=int32  SampleTime=-1
  Constant5 : Constant  Value=0  OutDataTypeStr=int32  SampleTime=-1
  Constant7 : Constant  Value=00000000000001  OutDataTypeStr=int32  SampleTime=-1
  Constant8 : Constant  Value=00000000000000  OutDataTypeStr=int32  SampleTime=-1
  Delay2 : Delay  DelayLength=1  InitialCondition=0
  Delay3 : Delay  DelayLength=1  InitialCondition=0
  Divide : Product  Inputs=***
  Divide1 : Product  Inputs=***
  Edge Detector : powerlib_meascontrol/Logic/Edge Detector  model=Rising  ic=0  Ts=-1
      settings: SourceProductBaseCode=PS
  Edge Detector2 : powerlib_meascontrol/Logic/Edge Detector  model=Rising  ic=0  Ts=-1
      settings: SourceProductBaseCode=PS
  GreaterThan : RelationalOperator  OutDataTypeStr=boolean  RndMeth=Simplest
  GreaterThan1 : RelationalOperator  Operator=<=  OutDataTypeStr=boolean  RndMeth=Simplest
  GreaterThan2 : RelationalOperator  Operator=<  OutDataTypeStr=boolean  RndMeth=Simplest
  GreaterThan3 : RelationalOperator  Operator=>  OutDataTypeStr=boolean  RndMeth=Simplest
  HystSelection1 : InportShadow  Port=4
  Input 1 : InportShadow
  Input 2 : InportShadow
  Less Than : RelationalOperator  Operator=<  OutDataTypeStr=boolean  RndMeth=Simplest
  LowerThd1 : InportShadow  Port=3
  LowerTrhd1 : InportShadow  Port=3
  Min : MinMax  Inputs=2
  Min1 : MinMax  Inputs=2
  Multiport Switch : MultiPortSwitch  Inputs=4
  Multiport Switch1 : MultiPortSwitch  Inputs=4
  RelHyst1 : InportShadow  Port=6
  Sum : Sum
  Sum2 : Sum
  Sum3 : Sum  Inputs=|++
  Sum4 : Sum  Inputs=+-
  Sum5 : Sum
  Switch{1..6} (6 alike) : Switch  Criteria=u2 > Threshold
  UpperThd1 : InportShadow  Port=2
  UpperTrhd1 : InportShadow  Port=2
  "Output " : Outport
  ErrorCode : Outport  Port=2
  wires:
  Sum3/1 -> Switch3/3
  Constant5/1 -> Switch3/1
  [improper] -> Switch3/2
  Switch3/1 -> "Output "/1
  LowerTrhd1/1 -> Less Than/2
  UpperTrhd1/1 -> Less Than/1
  Delay2/1 -> Switch6/3
  Delay3/1 -> Switch5/3
  Constant3/1 -> Switch6/1
  Constant1/1 -> Switch5/1
  GreaterThan2/1 -> Switch5/2
  LowerThd1/1 -> Sum5/2
  Multiport Switch1/1 -> Sum5/1
  Sum5/1 -> GreaterThan3/2
  UpperThd1/1 -> Sum4/1
  Multiport Switch/1 -> Sum4/2
  Sum4/1 -> GreaterThan2/2
  Switch1/1 -> Sum3/2, Delay2/1
  GreaterThan3/1 -> Switch6/2
  Switch6/1 -> Switch1/3
  Edge Detector2/1 -> Switch1/2
  GreaterThan1/1 -> Edge Detector2/1
  Input 2/1 -> GreaterThan3/1
  Sum2/1 -> Multiport Switch1/5
  [RelHysvalue1] -> Min1/1, Multiport Switch1/4, Sum2/2
  AbsHyst/1 -> Multiport Switch1/3, Min1/2, Sum2/1
  Min1/1 -> Multiport Switch1/2
  HystSelection1/1 -> Multiport Switch1/1
  Divide1/1 -> [RelHysvalue1]
  Constant2/1 -> Divide1/1
  RelHyst/1 -> Divide1/2
  RelHyst1/1 -> Divide/3
  Constant/1 -> Divide/2
  Switch4/1 -> Sum3/1, Delay3/1
  Switch5/1 -> Switch4/3
  Edge Detector/1 -> Switch4/2
  Constant10/1 -> Switch4/1
  Input 1/1 -> GreaterThan2/1
  Min/1 -> Multiport Switch/2
  Divide/1 -> [RelHysvalue]
  Sum/1 -> Multiport Switch/5
  [RelHysvalue] -> Multiport Switch/4, Sum/2, Min/1
  AbsHyst1/1 -> Multiport Switch/3, Sum/1, Min/2
  HystSelection/1 -> Multiport Switch/1
  LowerTrhd/1 -> GreaterThan1/2, Divide1/3
  UpperTrhd/1 -> GreaterThan/2, Divide/1
  "Input "/1 -> GreaterThan1/1, GreaterThan/1
  GreaterThan/1 -> Edge Detector/1
  Constant4/1 -> Switch1/1
  Constant7/1 -> Switch2/1
  Constant8/1 -> Switch2/3
  Less Than/1 -> Switch2/2, [improper]
  Switch2/1 -> ErrorCode/1

== system ESSLibrary/PFReference_P/If Action Subsystem/Safe Divider/Subsystem ==
  Numerator : Inport  OutDataTypeStr=double
  Denominator : Inport  Port=2  OutDataTypeStr=double
  Action Port : ActionPort
  Constant1 : Constant  OutDataTypeStr=int64  SampleTime=-1
  Constant11 : Constant  SampleTime=-1
  Constant2 : Constant  Value=0  OutDataTypeStr=int64  SampleTime=-1
  Divide8 : Product  Inputs=*/
  NOT : Logic  Operator=NOT  IconShape=distinctive  AllPortsSameDT=off  OutDataTypeStr=boolean
  NOT1 : Logic  Operator=NOT  IconShape=distinctive  AllPortsSameDT=off  OutDataTypeStr=boolean
  Subsystem21 : Subsystem
  Switch1 : Switch  Criteria=u2 ~= 0
  Switch11 : Switch  Criteria=u2 ~= 0
  Quality : Outport  OutDataTypeStr=boolean
  Out : Outport  Port=2  OutDataTypeStr=double
  ErrorCode : Outport  Port=3  OutDataTypeStr=int64
  wires:
  [Quality2] -> Quality/1
  Constant2/1 -> Switch1/1
  Switch11/1 -> Out/1
  Subsystem21/2(Quality) -> [Quality2]
  Constant11/1 -> Switch11/3
  Subsystem21/1(Divisor) -> [Divisor]
  Numerator/1 -> Divide8/1
  Divide8/1 -> Switch11/1
  [Quality2] -> NOT/1
  [Divisor] -> Divide8/2
  Denominator/1 -> Subsystem21/1(Denominator)
  Constant1/1 -> Switch1/3
  Switch1/1 -> ErrorCode/1
  [Quality2] -> NOT1/1
  NOT/1 -> Switch11/2
  NOT1/1 -> Switch1/2

== system ESSLibrary/PFReference_P/If Action Subsystem/Safe Divider/Subsystem1 ==
  In1 : Inport  OutDataTypeStr=double
  Action Port : ActionPort
  Constant1 : Constant  Value=9  OutDataTypeStr=int64  SampleTime=-1
  Constant11 : Constant  Value=0  OutDataTypeStr=boolean  SampleTime=-1
  Out3 : Outport  OutDataTypeStr=boolean
  Out4 : Outport  Port=2  OutDataTypeStr=double
  Out5 : Outport  Port=3  OutDataTypeStr=int64
  wires:
  Constant1/1 -> Out5/1
  Constant11/1 -> Out3/1
  In1/1 -> Out4/1

== system ESSLibrary/QReference_PF/If Action Subsystem/Subsystem1/Safe Divider ==
  Enable : Inport  OutDataTypeStr=boolean
  Numerator : Inport  Port=2  OutDataTypeStr=double
  Denominator : Inport  Port=3  OutDataTypeStr=double
  Abs : Abs
  If : If  IfExpression=u1 ~= 0
  Subsystem : Subsystem
  Subsystem1 : Subsystem
  Switch1 : Switch  Criteria=u2 ~= 0
  Switch6 : Switch  Criteria=u2 > Threshold
  Switch7 : Switch  Criteria=u2 > Threshold
  Switch8 : Switch  Criteria=u2 > Threshold
  Quotient : Outport  OutDataTypeStr=double
  Quality : Outport  Port=2  OutDataTypeStr=boolean
  ErrorCode : Outport  Port=3  OutDataTypeStr=int64
  wires:
  If/2 -> Subsystem1/Action
  [Quotient] -> Switch1/2, Switch1/1
  Switch6/1 -> Quality/1
  [DivErrorCode] -> Switch8/1
  Subsystem1/3(Out5) -> [DivErrorCodeD]
  Switch8/1 -> ErrorCode/1
  Subsystem/2(Out) -> [Quotient]
  [QuotientD] -> Switch7/3
  Denominator/1 -> [Denom]
  Switch7/1 -> Quotient/1
  [DivErrorCodeD] -> Switch8/3
  Subsystem1/1(Out3) -> [QualityD]
  Switch1/1 -> Switch7/1
  Subsystem/1(Quality) -> [Quality]
  If/1 -> Subsystem/Action
  Subsystem1/2(Out4) -> [QuotientD]
  [Denom] -> Subsystem/2(Denominator)
  Numerator/1 -> [Num]
  Subsystem/3(ErrorCode) -> [DivErrorCode]
  [Quotient] -> Abs/1
  [Num] -> Subsystem1/1(In1)
  [QualityD] -> Switch6/3
  Enable/1 -> If/1, Switch6/2, Switch7/2, Switch8/2
  Abs/1 -> Switch1/3
  [Num] -> Subsystem/1(Numerator)
  [Quality] -> Switch6/1

== system ESSLibrary/SoCManagement/IfActionSubsystem/Comparator/Basic alarm ver2.0 ==
  Enable/disable : Inport  OutDataTypeStr=boolean
  "Input " : Inport  Port=2
  UpperTrhd : Inport  Port=3
  LowerTrhd : Inport  Port=4
  HystSelection : Inport  Port=5  OutDataTypeStr=int32
  AbsHyst : Inport  Port=6
  RelHyst : Inport  Port=7
  Enable/disable1 : InportShadow  OutDataTypeStr=boolean
  Enabled Subsystem : Subsystem  TreatAsAtomicUnit=on
  Enabled Subsystem1 : Subsystem  TreatAsAtomicUnit=on
  If : If  IfExpression=u1 ~=0
  Switch : Switch  Criteria=u2 > Threshold
  Switch1 : Switch  Criteria=u2 > Threshold
  Switch3 : Switch  Criteria=u2 > Threshold
  MaxLimitCrossed : Outport  OutDataTypeStr=boolean
  MinLimitCrossed : Outport  Port=2  OutDataTypeStr=boolean
  ErrorCode : Outport  Port=3  OutDataTypeStr=int64
  wires:
  Switch3/1 -> ErrorCode/1
  Switch1/1 -> MinLimitCrossed/1
  [Else_MinLimitCrossed] -> Switch1/3
  [If_MinLimitCrossed] -> Switch1/1
  Enabled Subsystem/3(MinLimitCrossed) -> [Else_MinLimitCrossed]
  Enabled Subsystem1/2(MinLimitCrossed) -> [If_MinLimitCrossed]
  HystSelection/1 -> Enabled Subsystem1/4(HystSelection)
  RelHyst/1 -> Enabled Subsystem1/6(RelHyst)
  AbsHyst/1 -> Enabled Subsystem1/5(AbsHyst)
  LowerTrhd/1 -> Enabled Subsystem1/3(LowerTrhd)
  UpperTrhd/1 -> Enabled Subsystem1/2(UpperTrhd)
  "Input "/1 -> Enabled Subsystem1/1("Input ")
  Enable/disable1/1 -> Switch/2, Switch1/2, Switch3/2
  [Else_MaxLimitCrossed] -> Switch/3
  Switch/1 -> MaxLimitCrossed/1
  Enabled Subsystem1/1(MaxLimitCrossed) -> [If_MaxLimitCrossed]
  [Else_Errorcode] -> Switch3/3
  [If_Errorcode] -> Switch3/1
  [If_MaxLimitCrossed] -> Switch/1
  Enabled Subsystem/1("MaxLimitCrossed ") -> [Else_MaxLimitCrossed]
  Enabled Subsystem/2(ErrorCode) -> [Else_Errorcode]
  Enabled Subsystem1/3(ErrorCode) -> [If_Errorcode]
  If/1 -> Enabled Subsystem1/Action
  If/2 -> Enabled Subsystem/Action
  Enable/disable/1 -> If/1

== system ESSLibrary/Dispatch/IfActionSubsystem/PrioritySelector/ActivePowerPriority/ActivePowerPriority_NoPQCurve ==
  ActivePowerCalc : Inport
  ReactivePowerCalc : Inport  Port=2
  ECPAppPow : Inport  Port=3
  EnablePFLimit : Inport  Port=4
  PFOperMax : Inport  Port=5
  PFOperMin : Inport  Port=6
  Action Port : ActionPort  ActionPortLabel=else
  ActivePowerPriority_NoPQCurve : MATLAB Function  TreatAsAtomicUnit=on
  ActivePowerOut : Outport
  ReactivePowerOut : Outport  Port=2
  wires:
  ActivePowerCalc/1 -> ActivePowerPriority_NoPQCurve/1(ActivePowerCalc)
  ReactivePowerCalc/1 -> ActivePowerPriority_NoPQCurve/2(ReactivePowerCalc)
  ECPAppPow/1 -> ActivePowerPriority_NoPQCurve/3(ECPAppPow)
  EnablePFLimit/1 -> ActivePowerPriority_NoPQCurve/4(EnablePFLimit)
  PFOperMax/1 -> ActivePowerPriority_NoPQCurve/5(PFOperMax)
  PFOperMin/1 -> ActivePowerPriority_NoPQCurve/6(PFOperMin)
  ActivePowerPriority_NoPQCurve/1(ActivePowerOut) -> ActivePowerOut/1
  ActivePowerPriority_NoPQCurve/2(ReactivePowerOut) -> ReactivePowerOut/1

== system ESSLibrary/Dispatch/IfActionSubsystem/PrioritySelector/ActivePowerPriority/ActivePowerPriority_PQCurve ==
  Pcapability1 : Inport
  Pcapability2 : Inport  Port=2
  Pcapability3 : Inport  Port=3
  Pcapability4 : Inport  Port=4
  Pcapability5 : Inport  Port=5
  Pcapability6 : Inport  Port=6
  Pcapability7 : Inport  Port=7
  Pcapability8 : Inport  Port=8
  Qcapability1 : Inport  Port=9
  Qcapability2 : Inport  Port=10
  Qcapability3 : Inport  Port=11
  Qcapability4 : Inport  Port=12
  Qcapability5 : Inport  Port=13
  Qcapability6 : Inport  Port=14
  Qcapability7 : Inport  Port=15
  Qcapability8 : Inport  Port=16
  ECPAppPow : Inport  Port=17
  EnablePFLimit : Inport  Port=18
  PFOperMax : Inport  Port=19
  PFOperMin : Inport  Port=20
  ActivePowerCalc : Inport  Port=21
  ReactivePowerCalc : Inport  Port=22
  Action Port : ActionPort  ActionPortLabel=if(u1 == 1)
  ActivePowerEvaluator : MATLAB Function  TreatAsAtomicUnit=on
  ECPAppPow1 : InportShadow  Port=17
  PCapability Calculator : Subsystem
  Pcapability1_ : InportShadow
  Pcapability2_ : InportShadow  Port=2
  Pcapability3_ : InportShadow  Port=3
  Pcapability4_ : InportShadow  Port=4
  Pcapability5_ : InportShadow  Port=5
  Pcapability6_ : InportShadow  Port=6
  Pcapability7_ : InportShadow  Port=7
  Pcapability8_ : InportShadow  Port=8
  QCapabilityCalculator : Subsystem
  ReactivePowerEvaluator : MATLAB Function  TreatAsAtomicUnit=on
  ActivePowerOut : Outport
  ReactivePowerOut : Outport  Port=2
  wires:
  Pcapability1/1 -> PCapability Calculator/1(input1)
  Pcapability2/1 -> PCapability Calculator/2(input2)
  Pcapability3/1 -> PCapability Calculator/3(input3)
  Pcapability4/1 -> PCapability Calculator/4(input4)
  Pcapability5/1 -> PCapability Calculator/5(input5)
  Pcapability6/1 -> PCapability Calculator/6(input6)
  Pcapability7/1 -> PCapability Calculator/7(input7)
  Pcapability8/1 -> PCapability Calculator/8(input8)
  Pcapability1_/1 -> QCapabilityCalculator/1(X1)
  Qcapability1/1 -> QCapabilityCalculator/2(Y1)
  Pcapability2_/1 -> QCapabilityCalculator/3(X2)
  Qcapability2/1 -> QCapabilityCalculator/4(Y2)
  Pcapability3_/1 -> QCapabilityCalculator/5(X3)
  Qcapability3/1 -> QCapabilityCalculator/6(Y3)
  Pcapability4_/1 -> QCapabilityCalculator/7(X4)
  Qcapability4/1 -> QCapabilityCalculator/8(Y4)
  Pcapability5_/1 -> QCapabilityCalculator/9(X5)
  Qcapability5/1 -> QCapabilityCalculator/10(Y5)
  Pcapability6_/1 -> QCapabilityCalculator/11(X6)
  Qcapability6/1 -> QCapabilityCalculator/12(Y6)
  Pcapability7_/1 -> QCapabilityCalculator/13(X7)
  Qcapability7/1 -> QCapabilityCalculator/14(Y7)
  Pcapability8_/1 -> QCapabilityCalculator/15(X8)
  Qcapability8/1 -> QCapabilityCalculator/16(Y8)
  [ActivePowerOut] -> QCapabilityCalculator/17(input)
  QCapabilityCalculator/1(YMax) -> [MaxQ]
  QCapabilityCalculator/2(YMin) -> [MinQ]
  PCapability Calculator/1(Maximum) -> [MaxP]
  PCapability Calculator/2(Minimum) -> [MinP]
  [MaxP] -> ActivePowerEvaluator/2(MaxP_PQCurve)
  [MinP] -> ActivePowerEvaluator/3(MinP_PQCurve)
  ECPAppPow/1 -> ActivePowerEvaluator/4(ECPAppPow)
  ActivePowerCalc/1 -> ActivePowerEvaluator/1(ActivePowerCalc)
  ActivePowerEvaluator/1(ActivePowerOut) -> [ActivePowerOut]
  [ActivePowerOut] -> ActivePowerOut/1
  [MinQ] -> ReactivePowerEvaluator/4(MinQ_PQCurve)
  [MaxQ] -> ReactivePowerEvaluator/3(MaxQ_PQCurve)
  ReactivePowerCalc/1 -> ReactivePowerEvaluator/1(ReactivePowerCalc)
  [ActivePowerOut] -> ReactivePowerEvaluator/2(ActivePowerCalc)
  ECPAppPow1/1 -> ReactivePowerEvaluator/5(ECPAppPow)
  EnablePFLimit/1 -> ReactivePowerEvaluator/6(EnablePFLimit)
  PFOperMax/1 -> ReactivePowerEvaluator/7(PFOperMax)
  PFOperMin/1 -> ReactivePowerEvaluator/8(PFOperMin)
  ReactivePowerEvaluator/1(ReactivePowerOut) -> [ReactivePowerOut]
  [ReactivePowerOut] -> ReactivePowerOut/1

== system ESSLibrary/Dispatch/IfActionSubsystem/PrioritySelector/ReactivePowerPriority/ReactivePowerPriority_NoPQCurve ==
  ActivePowerCalc : Inport
  ReactivePowerCalc : Inport  Port=2
  ECPAppPow : Inport  Port=3
  EnablePFLimit : Inport  Port=4
  PFOperMax : Inport  Port=5
  PFOperMin : Inport  Port=6
  Action Port : ActionPort
  ReactivePowerPriority_NoPQCurve : MATLAB Function  TreatAsAtomicUnit=on
  ActivePowerOut : Outport
  ReactivePowerOut : Outport  Port=2
  wires:
  ActivePowerCalc/1 -> ReactivePowerPriority_NoPQCurve/1(ActivePowerCalc)
  ReactivePowerCalc/1 -> ReactivePowerPriority_NoPQCurve/2(ReactivePowerCalc)
  ECPAppPow/1 -> ReactivePowerPriority_NoPQCurve/3(ECPAppPow)
  EnablePFLimit/1 -> ReactivePowerPriority_NoPQCurve/4(EnablePFLimit)
  PFOperMax/1 -> ReactivePowerPriority_NoPQCurve/5(PFOperMax)
  PFOperMin/1 -> ReactivePowerPriority_NoPQCurve/6(PFOperMin)
  ReactivePowerPriority_NoPQCurve/1(ActivePowerOut) -> ActivePowerOut/1
  ReactivePowerPriority_NoPQCurve/2(ReactivePowerOut) -> ReactivePowerOut/1

== system ESSLibrary/Dispatch/IfActionSubsystem/PrioritySelector/ReactivePowerPriority/ReactivePowerPriority_PQCurve ==
  Pcapability1 : Inport
  Pcapability2 : Inport  Port=2
  Pcapability3 : Inport  Port=3
  Pcapability4 : Inport  Port=4
  Pcapability5 : Inport  Port=5
  Pcapability6 : Inport  Port=6
  Pcapability7 : Inport  Port=7
  Pcapability8 : Inport  Port=8
  Qcapability1 : Inport  Port=9
  Qcapability2 : Inport  Port=10
  Qcapability3 : Inport  Port=11
  Qcapability4 : Inport  Port=12
  Qcapability5 : Inport  Port=13
  Qcapability6 : Inport  Port=14
  Qcapability7 : Inport  Port=15
  Qcapability8 : Inport  Port=16
  ECPAppPow : Inport  Port=17
  EnablePFLimit : Inport  Port=18
  PFOperMax : Inport  Port=19
  PFOperMin : Inport  Port=20
  ActivePowerCalc : Inport  Port=21
  ReactivePowerCalc : Inport  Port=22
  Action Port : ActionPort
  ActivePowerEvaluator1 : MATLAB Function  TreatAsAtomicUnit=on
  ECPAppPow1 : InportShadow  Port=17
  QCapability Calculator : Subsystem
  QCapabilityCalculator : Subsystem
  Qcapability1_ : InportShadow  Port=9
  Qcapability2_ : InportShadow  Port=10
  Qcapability3_ : InportShadow  Port=11
  Qcapability4_ : InportShadow  Port=12
  Qcapability5_ : InportShadow  Port=13
  Qcapability6_ : InportShadow  Port=14
  Qcapability7_ : InportShadow  Port=15
  Qcapability8_ : InportShadow  Port=16
  ReactivePowerEvaluator : MATLAB Function  TreatAsAtomicUnit=on
  ActivePowerOut : Outport
  ReactivePowerOut : Outport  Port=2
  wires:
  [ReactivePowerOut] -> QCapabilityCalculator/17(input)
  QCapabilityCalculator/1(YMax) -> [MaxP]
  QCapabilityCalculator/2(YMin) -> [MinP]
  QCapability Calculator/1(Maximum) -> [MaxQ]
  QCapability Calculator/2(Minimum) -> [MinQ]
  [MaxQ] -> ReactivePowerEvaluator/2(MaxQ_PQCurve)
  [MinQ] -> ReactivePowerEvaluator/3(MinQ_PQCurve)
  ECPAppPow/1 -> ReactivePowerEvaluator/4(ECPAppPow)
  [ActivePowerOut] -> ActivePowerOut/1
  [MinP] -> ActivePowerEvaluator1/4(MinP_PQCurve)
  [MaxP] -> ActivePowerEvaluator1/3(MaxP_PQCurve)
  [ReactivePowerOut] -> ActivePowerEvaluator1/2(ActivePowerCalc)
  ECPAppPow1/1 -> ActivePowerEvaluator1/5(ECPAppPow)
  EnablePFLimit/1 -> ActivePowerEvaluator1/6(EnablePFLimit)
  PFOperMax/1 -> ActivePowerEvaluator1/7(PFOperMax)
  PFOperMin/1 -> ActivePowerEvaluator1/8(PFOperMin)
  [ReactivePowerOut] -> ReactivePowerOut/1
  Qcapability1_/1 -> QCapability Calculator/1(input1)
  Qcapability2_/1 -> QCapability Calculator/2(input2)
  Qcapability3_/1 -> QCapability Calculator/3(input3)
  Qcapability4_/1 -> QCapability Calculator/4(input4)
  Qcapability5_/1 -> QCapability Calculator/5(input5)
  Qcapability6_/1 -> QCapability Calculator/6(input6)
  Qcapability7_/1 -> QCapability Calculator/7(input7)
  Qcapability8_/1 -> QCapability Calculator/8(input8)
  ReactivePowerCalc/1 -> ReactivePowerEvaluator/1(ReactivePowerCalc)
  ReactivePowerEvaluator/1(ReactivePowerOut) -> [ReactivePowerOut]
  Qcapability1/1 -> QCapabilityCalculator/1(X1)
  Pcapability1/1 -> QCapabilityCalculator/2(Y1)
  Qcapability2/1 -> QCapabilityCalculator/3(X2)
  Pcapability2/1 -> QCapabilityCalculator/4(Y2)
  Qcapability3/1 -> QCapabilityCalculator/5(X3)
  Pcapability3/1 -> QCapabilityCalculator/6(Y3)
  Qcapability4/1 -> QCapabilityCalculator/7(X4)
  Pcapability4/1 -> QCapabilityCalculator/8(Y4)
  Qcapability5/1 -> QCapabilityCalculator/9(X5)
  Pcapability5/1 -> QCapabilityCalculator/10(Y5)
  Qcapability6/1 -> QCapabilityCalculator/11(X6)
  Pcapability6/1 -> QCapabilityCalculator/12(Y6)
  Qcapability7/1 -> QCapabilityCalculator/13(X7)
  Pcapability7/1 -> QCapabilityCalculator/14(Y7)
  Qcapability8/1 -> QCapabilityCalculator/15(X8)
  Pcapability8/1 -> QCapabilityCalculator/16(Y8)
  ActivePowerCalc/1 -> ActivePowerEvaluator1/1(ReactivePowerCalc)
  ActivePowerEvaluator1/1(ActivePowerOut) -> [ActivePowerOut]

== system ESSLibrary/OperationModeSelector/IfAction Subsystem/Comparator/Basic alarm ver2.0/Enabled Subsystem ==
  Action Port : ActionPort
  Constant3 : Constant  Value=0  OutDataTypeStr=boolean  SampleTime=-1
  "MaxLimitCrossed " : Outport
  ErrorCode : Outport  Port=2
  MinLimitCrossed : Outport  Port=3
  wires:
  Constant3/1 -> ErrorCode/1, MinLimitCrossed/1, "MaxLimitCrossed "/1
